simulink model "point_mass_test"  (R2021b)
settings: Solver=VariableStepAuto  StartTime=0.0  StopTime=50  RelTol=1e-3
StartFcn:
  | pint_mass_test
StopFcn:
  | plot_stuff
values from neighbouring files (symbols this model uses):
  A = sqrt(d*(d-a)*(d-b)*(d-c))    [dnMPC_test.m]
  C = 3003730.83469    [this workspace breakes the state change functions.mat]
  K = track(4)    [dbike_model.m]    (also in dnMPC_test.m = 4*A/(a*b*c); knState.m)
undefined symbols (not defined in the file or in its folder): B, D, x_init
libraries: mpclib x1
settings Model: Creator=PLASMINFORGE  LastModifiedBy=PLASMINFORGE

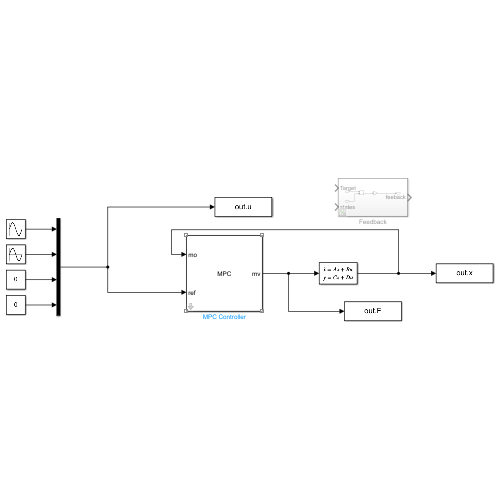
[thumbnail: Simulink's stored preview of the top-level diagram]
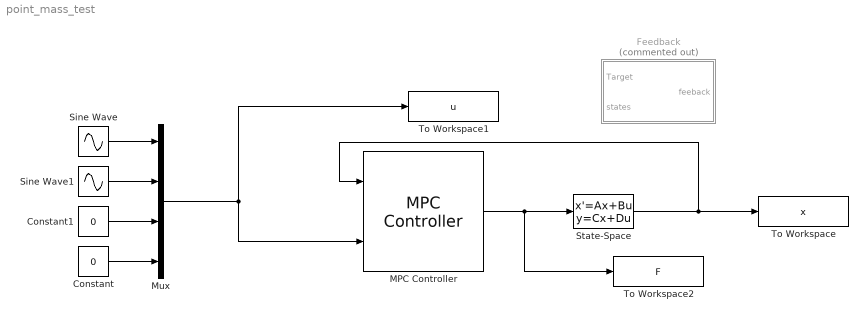
== system point_mass_test ==
  Constant : Constant  Value=0
  Constant1 : Constant  Value=0
  Feedback : Subsystem  Commented=on
  MPC Controller : mpclib/MPC Controller  SCDEnableBlockLinearizationSpecification=on  mpcobj=mpc1  is_multiple=0  enable_value=0  return_u0=off  updateMPCinCallerWorkspace=on  md_inport=off  mv_inport=off  uref_inport=off  return_cost=off  return_mvseq=off  return_qpstatus=off  return_xseq=off  return_state=off  return_ovseq=off  state_inport=off  umin_inport=off  umax_inport=off  ymin_inport=off  ymax_inport=off  cc_inport=off  ywt_inport=off  uwt_inport=off  duwt_inport=off  rhoeps_inport=off  pm_inport=off  MaximumP=10  HorizonChoice=FixedHorizon  n_ts=0.1  n_p=30  n_mv=2  n_md=0  n_ud=0  n_mo=4  n_uo=0  BlockDataType=double  SampleTimeInherited=off  switch_inport=off
  Mux : Mux
  Sine Wave : Sin  SampleTime=0
  Sine Wave1 : Sin  Phase=pi/2  SampleTime=0
  State-Space : StateSpace  A=A  B=B  C=C  D=D  InitialCondition=x_init
  To Workspace : ToWorkspace  VariableName=x  SampleTime=-1
      settings: Save2DSignal=2-D array (concatenate along first dimension)
  To Workspace1 : ToWorkspace  VariableName=u  SampleTime=-1
      settings: Save2DSignal=2-D array (concatenate along first dimension)
  To Workspace2 : ToWorkspace  VariableName=F  SampleTime=-1
      settings: Save2DSignal=2-D array (concatenate along first dimension)
  wires:
  State-Space/1 -> MPC Controller/1, To Workspace/1
  Mux/1 -> To Workspace1/1, MPC Controller/2
  Constant/1 -> Mux/4
  Constant1/1 -> Mux/3
  Sine Wave1/1 -> Mux/2
  Sine Wave/1 -> Mux/1
  MPC Controller/1 -> To Workspace2/1, State-Space/1

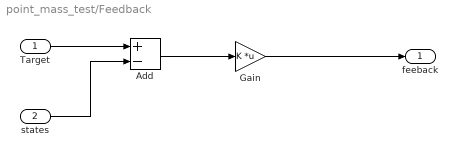
== system point_mass_test/Feedback ==
  Target : Inport
  states : Inport  Port=2
  Add : Sum  Inputs=+-
  Gain : Gain  Gain=K  Multiplication=Matrix(K*u)
  feeback : Outport
  wires:
  Add/1 -> Gain/1
  Target/1 -> Add/1
  Gain/1 -> feeback/1
  states/1 -> Add/2
